simulink model "modele2"  (R2021a)
settings: Solver=VariableStepAuto  StartTime=0.0  StopTime=20  RelTol=10e-8
values from neighbouring files (symbols this model uses):
  A_L = 1    [etablissement_variables.m]
  A_S = 1    [etablissement_variables.m]
  c = 2000.*[1 1 1 1]    [etablissement_variables.m]
  C_x = 1    [etablissement_variables.m]
  Cte_1 = 1    [etablissement_variables.m]
  Cte_2 = 1    [etablissement_variables.m]
  Cte_3 = 1    [etablissement_variables.m]
  Cte_4 = 1    [etablissement_variables.m]
  d_f = 1    [etablissement_variables.m]
  d_r = 1    [etablissement_variables.m]
  g = 9.81    [etablissement_variables.m]
  h = 1    [etablissement_variables.m]
  I = [2 0 0; 0 3 0; 0 0 3]    [etablissement_variables.m]
  J = [1 1 1 1]    [etablissement_variables.m]
  k = 30000.*[1 1 1 1]    [etablissement_variables.m]
  L = l_r+l_f    (= 2)    [etablissement_variables.m]
  l_f = L-l_r    [calcul_N.m]    (also in etablissement_variables.m = 1)
  l_r = 1    [etablissement_variables.m]
  M = 400    [etablissement_variables.m]
  m = M/4.*[l_f/L l_f/L l_r/L l_r/L]    [etablissement_variables.m]
  R = [1 1 1 1]    [etablissement_variables.m]
  rho = 1    [etablissement_variables.m]
undefined symbols (not defined in the file or in its folder): calcul_adherence, calcul_delta, calcul_Fcz, calcul_forceaero, calcul_forces, calcul_forcesprojetees, calcul_lambda, calcul_matriceforces, calcul_matricemoments, calcul_N, calcul_omega, calcul_retourvitesse, calcul_rotaroute, calcul_rotation, calcul_secondterme, calcul_slipangle, calcul_vitessesroues, projection
libraries: dsparch4 x3, slpidlib x2
settings Model: PauseTimes=0.1  Creator=TP-EEA  LastModifiedBy=TP-EEA
settings DebuggingCC: SignalInfNanChecking=error
settings ModelReferenceCC: ModelReferenceMinAlgLoopOccurrences=on

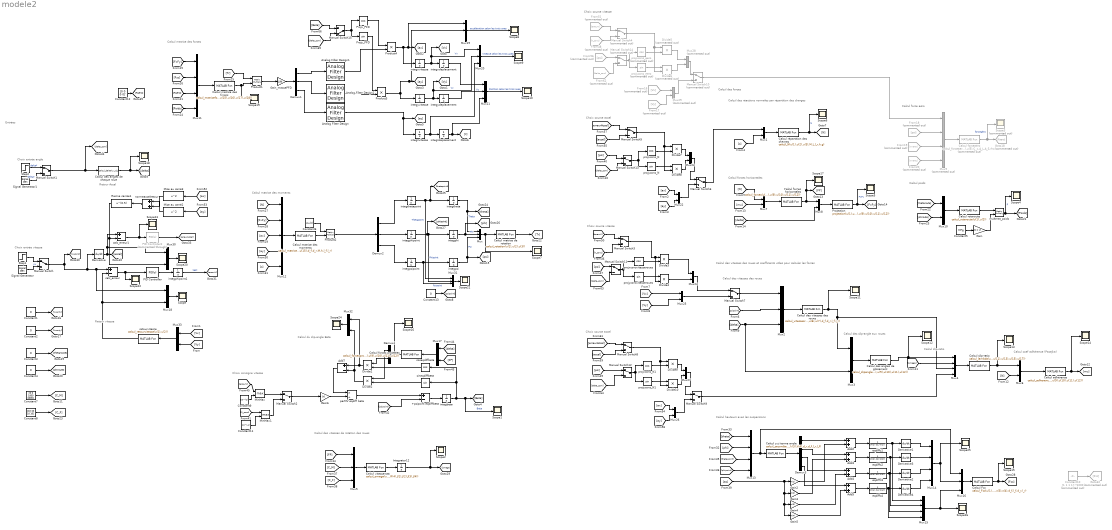
== system modele2 ==
  note: Choix consigne vitesse
  note: Choix entrée vitesse
  note: Choix entrée angle
  note: Choix source accel
  note: Calcul du slip-angle Beta
  note: Calcul des vitesses de rotation des roues
  note: Calcul matrice des forces
  note: Calcul poids
  note: Calcul force aéro
  note: Calcul des forces
  note: Calcul forces horizontales
  note: Calcul des vitesses des roues et coefficients utiles pour calculer les forces
  note: Calcul coef adhérence (Pacejka)
  note: Calcul slip-ratio
  note: Calcul des slip-angle aux roues
  note: Calcul des vitesses des roues
  note: Calcul des réactions normales par répartition des charges
  note: Retour vitesse
  note: Entrées
  note: Calcul matrice des moments
  note: Calcul hauteurs avec les suspensions
  note: Retour Accel
  note: Choix source vitesse
  note: Choix source accel
  note: Choix source vitesse
  +psipoint eqdiffbeta : Sum  Inputs=+-
  Add{2..5} (4 alike) : Sum
  Add7 : Sum  Inputs=+-
  Analog Filter Design : dsparch4/Analog Filter Design  method=Butterworth  filttype=Lowpass  N=4  Wlo=20  Whi=80  Rp=2  Rs=40
  Analog Filter Design1 : dsparch4/Analog Filter Design  method=Butterworth  filttype=Lowpass  N=4  Wlo=20  Whi=80  Rp=2  Rs=40
  Analog Filter Design2 : dsparch4/Analog Filter Design  method=Butterworth  filttype=Lowpass  N=4  Wlo=20  Whi=80  Rp=2  Rs=40
  Calcul Fzc : MATLABFcn  MATLABFcn=calcul_Fcz(u(1),u(2),u(3),u(4),u(5),u(6),u(7),u(8),u(9),u(10),u(11),u(12),k(1),k(2),k(3),k(4),c(1),c(2),c(3),c(4),d_f,l_f,d_r,l_r)  OutputDimensions=4
  Calcul adhérence : MATLABFcn  MATLABFcn=calcul_adherence(u(1),u(2),u(3),u(4),u(5),u(6),u(7),u(8),Cte_1,Cte_2,Cte_3,Cte_4,u(9),u(10),u(11),u(12))  OutputDimensions=4*2
  Calcul des angles de chaque roue : MATLABFcn  MATLABFcn=calcul_delta(u,L,d_f)  OutputDimensions=4
  Calcul des angles de glissement : MATLABFcn  MATLABFcn=calcul_slipangle(u(1),u(2),u(3),u(4),u(5),u(6),u(7),u(8),u(9),u(10),u(11),u(12))  OutputDimensions=4
  Calcul des vitesses des roues : MATLABFcn  MATLABFcn=calcul_vitessesroues(u(1),u(2),u(3),u(4),u(5),u(6),u(7),d_f,d_r,l_f,l_r)  OutputDimensions=4*2
  Calcul forceaéro : MATLABFcn  Commented=on  MATLABFcn=calcul_forceaero(u(1),u(2),u(3),u(4),u(5),C_x,A_L,A_S,rho)  OutputDimensions=3
  Calcul forces horizontales : MATLABFcn  MATLABFcn=calcul_forces(u(1),u(2),u(3),u(4),u(5),u(6),u(7),u(8),u(9),u(10),u(11),u(12))  OutputDimensions=4*2
  Calcul forces projetées : MATLABFcn  MATLABFcn=calcul_forcesprojetees(u(1),u(2),u(3),u(4),u(5),u(6),u(7),u(8),u(9),u(10),u(11),u(12))  OutputDimensions=2  Output1D=off
  Calcul matrice de rotation : MATLABFcn  MATLABFcn=calcul_rotation(u(1),u(2),u(3))  OutputDimensions=[3 3]  Output1D=off
  Calcul matrice des forces : MATLABFcn  MATLABFcn=calcul_matriceforces(u(1),u(2),u(3),u(4),u(5),u(6),u(7),u(8),u(9),u(10),u(11),u(12),u(13),u(14),u(15),u(16),u(17),u(18))  OutputDimensions=[3 1]  Output1D=off
  Calcul matrice des moments : MATLABFcn  MATLABFcn=calcul_matricemoments(u(1),u(2),u(3),u(4),u(5),u(6),u(7),u(8),u(9),u(10),u(11),u(12),u(13),u(14),u(15),d_f,d_r,M,h,l_f,l_r)  OutputDimensions=[3 1]  Output1D=off
  Calcul rotaroute : MATLABFcn  MATLABFcn=calcul_rotaroute(u(1),u(2))  OutputDimensions=[3 3]  Output1D=off
  Calcul répartition des charges : MATLABFcn  MATLABFcn=calcul_N(u(1),u(2),u(3),M,L,l_r,h,g)  OutputDimensions=4
  Calcul slip-ratio : MATLABFcn  MATLABFcn=calcul_lambda(u(1),u(2),u(3),u(4),R(1),R(2),R(3),R(4),u(5),u(6),u(7),u(8),u(9),u(11),u(13),u(15),u(17))  OutputDimensions=4*2
  Calcul vitesserota : MATLABFcn  MATLABFcn=calcul_omega(u(1),u(2),u(3),u(4),u(5),u(6),u(7),u(8),u(9),u(10),u(11),u(12),u(13),u(14),u(15),u(16),R(1),R(2),R(3),R(4),J(1),J(2),J(3),J(4))  OutputDimensions=4
  Calcul z-zi terme angle : MATLABFcn  MATLABFcn=calcul_secondterme(u(1),u(2),u(3),u(4),c(1),c(2),c(3),c(4),k(1),k(2),k(3),k(4),d_r,d_f,l_r,l_f)  OutputDimensions=4
  Constant{1..4,13} (5 alike) : Constant  Value=0
  Constant10 : Constant  Commented=on  Value=[1 1 1 1]'.*1000  VectorParams1D=off
  Constant11 : Constant  Value=10^(-1)
  Constant12 : Constant  Value=[0 0 0 0]'
  Constant5 : Constant  Value=M*g  VectorParams1D=off
  Constant6 : Constant  Value=inv(I)
  Constant7 : Constant  Value=[0 0 1000 1000]
  Constant8 : Constant  Value=[10 10 10 10]
  Constant9 : Constant  Value=10^(-1)
  Demux1 : Demux  Outputs=3
  Demux2 : Demux  Outputs=3
  Demux3 : Demux
  Demux4 : Demux  Outputs=2
  Derivative{,1..4} (5 alike) : Derivative
  Divide{1..4,7..10} (8 alike) : Product  Inputs=**
  Divide5 : Product  Commented=on  Inputs=**
  Divide6 : Product  Commented=on  Inputs=**
  From16 : From  Commented=on  GotoTag=Vx
  From17 : From  Commented=on  GotoTag=Vy
  From18 : From  Commented=on  GotoTag=psi
  From19 : From  Commented=on  GotoTag=Vventx
  From20 : From  Commented=on  GotoTag=Vventy
  From48 : From  Commented=on  GotoTag=V_cons
  From51 : From  Commented=on  GotoTag=erreurV
  From56 : From  Commented=on  GotoTag=psi
  From62 : From  Commented=on  GotoTag=delta_com
  Gain : Gain  Gain=[0 0 1]'
  Gain2 : Gain  Gain=m(1)
  Gain3 : Gain  Gain=m(2)
  Gain4 : Gain  Gain=m(3)
  Gain5 : Gain  Gain=m(4)
  Gain6 : Gain  Gain=M
  Gain_massePFD : Gain  Gain=1/M
  Goto18 : Goto  Commented=on  GotoTag=Faero
  Goto32 : Goto  Commented=on  GotoTag=Fzc
  Integrator12 : Integrator
  Manual Switch{,1..3,5..9,11..13} (12 alike) : ManualSwitch
  Manual Switch10 : ManualSwitch  Commented=on
  Manual Switch14 : ManualSwitch  Commented=on
  Manual Switch15 : ManualSwitch  CurrentSetting=0
  Manual Switch4 : ManualSwitch  Commented=on
  MinMax : MinMax  Function=max  Inputs=2
  MinMax1 : MinMax  Function=max  Inputs=2
  Mise au carré2 : MATLABFcn  MATLABFcn=u^2
  Mise au carré3 : MATLABFcn  MATLABFcn=u^2
  Mux{,2,5,16,19..21,31} (8 alike) : Mux  Inputs=3
  Mux{1,3,6..8,10,17..18,22..27,30,32..33} (17 alike) : Mux  Inputs=2
  Mux{4,11,13..15} (5 alike) : Mux
  Mux12 : Mux  Inputs=5
  Mux28 : Mux  Commented=on  Inputs=2
  Mux29 : Mux  Commented=on  Inputs=2
  Mux9 : Mux  Commented=on
  PID Controller : slpidlib/PID Controller  Controller=PID  Form=Parallel  TimeDomain=Continuous-time  UseExternalTs=off  SampleTime=-1  IntegratorMethod=Forward Euler  FilterMethod=Forward Euler  ControllerParametersSource=internal  P=1  I=1000  D=0  UseFilter=on  N=100  TunerSelectOption=Transfer Function Based (PID Tuner App)  InitialConditionSource=internal  InitialConditionForIntegrator=0  InitialConditionForFilter=0  DifferentiatorICPrevScaledInput=0  ExternalReset=none  TrackingMode=off  Kt=1  LimitOutput=off  SatLimitsSource=internal  UpperSaturationLimit=inf  LowerSaturationLimit=-inf  LinearizeAsGain=on  AntiWindupMode=none  Kb=1  POutMin=[]  POutMax=[]  IOutMin=[]  IOutMax=[]  DOutMin=[]  DOutMax=[]  NOutMin=[]  NOutMax=[]  SumOutMin=[]  SumOutMax=[]  SaturationOutMin=[]  SaturationOutMax=[]  PParamMin=[]  PParamMax=[]  IParamMin=[]  IParamMax=[]  DParamMin=[]  DParamMax=[]  NParamMin=[]  NParamMax=[]  KbParamMin=[]  KbParamMax=[]  KtParamMin=[]  KtParamMax=[]  KbOutMin=[]  KbOutMax=[]  KtOutMin=[]  KtOutMax=[]  IntegratorOutMin=[]  IntegratorOutMax=[]  FilterOutMin=[]  FilterOutMax=[]  SumI1OutMin=[]  SumI1OutMax=[]  SumI2OutMin=[]  SumI2OutMax=[]  SumI3OutMin=[]  SumI3OutMax=[]  SumI4OutMin=[]  SumI4OutMax=[]  SumDOutMin=[]  SumDOutMax=[]  DifferentiatorOutMin=[]  DifferentiatorOutMax=[]  FilterDiffOutCoefMin=[]  FilterDiffOutCoefMax=[]  ReciprocalOutMin=[]  ReciprocalOutMax=[]  SumDenOutMin=[]  SumDenOutMax=[]  SumNumOutMin=[]  SumNumOutMax=[]  DivideOutMin=[]  DivideOutMax=[]  UdiffTsProdOutMin=[]  UdiffTsProdOutMax=[]  NTsProdOutMin=[]  NTsProdOutMax=[]  UintegralTsProdOutMin=[]  UintegralTsProdOutMax=[]  UngainTsProdOutMin=[]  UngainTsProdOutMax=[]  IntegratorContinuousStateAttributes=''  IntegratorStateMustResolveToSignalObject=off  IntegratorRTWStateStorageClass=Auto  FilterContinuousStateAttributes=''  FilterStateMustResolveToSignalObject=off  FilterRTWStateStorageClass=Auto  ParallelPVariant=InternalParameters  IdealPVariant=Disabled  IVariant=InternalParameters  DVariant=InternalParameters  IntegratorVariant=Continuous  SatVariant=Disabled  AWVariant=Passthrough  PCopyVariant=Disabled  TRVariant=Disabled  FdbkBlocksVariant=Forward  IdealPFdbkVariant=Disabled  SatFdbkVariant=Disabled  DerivativeFilterVariant=ContFilter  NVariant=InternalParameters  NCopyVariant=Disabled  FilterICVariant=InternalICsFilter  IntegratorICVariant=InternalICs  ExternalResetVariant=Disabled  TRSumVariant=Passthrough  SumFdbkVariant=Disabled  SumVariant=Sum_PID  TsampFilterVariant=InternalTs  TsampNgainVariant=Passthrough  TsampIntegralVariant=Passthrough  ExternalSaturationOutDataTypeStr=Inherit: Same as second input
  PID Controller2 : slpidlib/PID Controller  Commented=through  Controller=PID  Form=Parallel  TimeDomain=Continuous-time  UseExternalTs=off  SampleTime=-1  IntegratorMethod=Forward Euler  FilterMethod=Forward Euler  ControllerParametersSource=internal  P=1  I=1  D=0  UseFilter=on  N=100  TunerSelectOption=Transfer Function Based (PID Tuner App)  InitialConditionSource=internal  InitialConditionForIntegrator=0  InitialConditionForFilter=0  DifferentiatorICPrevScaledInput=0  ExternalReset=none  TrackingMode=off  Kt=1  LimitOutput=off  SatLimitsSource=internal  UpperSaturationLimit=inf  LowerSaturationLimit=-inf  LinearizeAsGain=on  AntiWindupMode=none  Kb=1  POutMin=[]  POutMax=[]  IOutMin=[]  IOutMax=[]  DOutMin=[]  DOutMax=[]  NOutMin=[]  NOutMax=[]  SumOutMin=[]  SumOutMax=[]  SaturationOutMin=[]  SaturationOutMax=[]  PParamMin=[]  PParamMax=[]  IParamMin=[]  IParamMax=[]  DParamMin=[]  DParamMax=[]  NParamMin=[]  NParamMax=[]  KbParamMin=[]  KbParamMax=[]  KtParamMin=[]  KtParamMax=[]  KbOutMin=[]  KbOutMax=[]  KtOutMin=[]  KtOutMax=[]  IntegratorOutMin=[]  IntegratorOutMax=[]  FilterOutMin=[]  FilterOutMax=[]  SumI1OutMin=[]  SumI1OutMax=[]  SumI2OutMin=[]  SumI2OutMax=[]  SumI3OutMin=[]  SumI3OutMax=[]  SumI4OutMin=[]  SumI4OutMax=[]  SumDOutMin=[]  SumDOutMax=[]  DifferentiatorOutMin=[]  DifferentiatorOutMax=[]  FilterDiffOutCoefMin=[]  FilterDiffOutCoefMax=[]  ReciprocalOutMin=[]  ReciprocalOutMax=[]  SumDenOutMin=[]  SumDenOutMax=[]  SumNumOutMin=[]  SumNumOutMax=[]  DivideOutMin=[]  DivideOutMax=[]  UdiffTsProdOutMin=[]  UdiffTsProdOutMax=[]  NTsProdOutMin=[]  NTsProdOutMax=[]  UintegralTsProdOutMin=[]  UintegralTsProdOutMax=[]  UngainTsProdOutMin=[]  UngainTsProdOutMax=[]  IntegratorContinuousStateAttributes=''  IntegratorStateMustResolveToSignalObject=off  IntegratorRTWStateStorageClass=Auto  FilterContinuousStateAttributes=''  FilterStateMustResolveToSignalObject=off  FilterRTWStateStorageClass=Auto  ParallelPVariant=InternalParameters  IdealPVariant=Disabled  IVariant=InternalParameters  DVariant=InternalParameters  IntegratorVariant=Continuous  SatVariant=Disabled  AWVariant=Passthrough  PCopyVariant=Disabled  TRVariant=Disabled  FdbkBlocksVariant=Forward  IdealPFdbkVariant=Disabled  SatFdbkVariant=Disabled  DerivativeFilterVariant=ContFilter  NVariant=InternalParameters  NCopyVariant=Disabled  FilterICVariant=InternalICsFilter  IntegratorICVariant=InternalICs  ExternalResetVariant=Disabled  TRSumVariant=Passthrough  SumFdbkVariant=Disabled  SumVariant=Sum_PID  TsampFilterVariant=InternalTs  TsampNgainVariant=Passthrough  TsampIntegralVariant=Passthrough  ExternalSaturationOutDataTypeStr=Inherit: Same as second input
  Product1 : Product  Multiplication=Matrix(*)
  Product2 : Product  Multiplication=Matrix(*)
  Product3 : Product
  Product4 : Product
  Projection : MATLABFcn  MATLABFcn=projection(u(1),u(2),u(3),u(4),u(5),u(6),u(7),u(8),u(9),u(10),u(11),u(12))  OutputDimensions=8
  Projx_PFD : Trigonometry  Operator=cos
  Projy_PFD : Trigonometry
  Racine carrée1 : MATLABFcn  MATLABFcn=u^(0.5)
  Scope{,1..2,4..26} (26 alike) : Scope
  Scope3 : Scope  Commented=on
  Signal Generator : SignalGenerator  Frequency=0.1  Units=rad/sec
  Signal Generator1 : SignalGenerator  Frequency=0.01  Units=rad/sec
  Step1 : Step  Time=0  After=10/3.6  SampleTime=0
  Step2 : Step  Time=0  After=0  SampleTime=0
  calc_erreur : Sum  Inputs=+-
  calc_erreur1 : Sum  Inputs=+-
  coseqdiffbeta : Trigonometry  Operator=cos
  eqdiffz1 : TransferFcn  Denominator=[m(1) c(1) k(1)]
  eqdiffz2 : TransferFcn  Denominator=[m(2) c(2) k(2)]
  eqdiffz3 : TransferFcn  Denominator=[m(3) c(3) k(3)]
  eqdiffz4 : TransferFcn  Denominator=[m(4) c(4) k(4)]
  integbeta : Integrator
  integphi : Integrator
  integphipoint : Integrator
  integphipoint1 : Integrator
  integpsi : Integrator
  integpsipoint : Integrator
  integtheta : Integrator
  integthetapoint : Integrator  InitialCondition=0.01
  integxdeplacement : Integrator
  integxvitesse : Integrator
  integydeplacement : Integrator
  integyvitesse : Integrator
  integzdeplacement : Integrator
  integzvitesse : Integrator
  multmat_poids : Product  Multiplication=Matrix(*)
  normeaccelretour : Sum
  parMV eqdiff beta : Product  Inputs=*/
  projxcons_N : Trigonometry  Operator=cos
  projxcons_N1 : Trigonometry  Operator=cos
  projxcons_aero : Trigonometry  Commented=on  Operator=cos
  projxconsvitesseroues : Trigonometry  Operator=cos
  projycons_N : Trigonometry
  projycons_N1 : Trigonometry
  projycons_aero : Trigonometry  Commented=on
  projyconsvitesseroues : Trigonometry
  retourvitesse : MATLABFcn  MATLABFcn=calcul_retourvitesse(u(1),u(2))  OutputDimensions=1
  sineqdiffbeta : Trigonometry
  wires:
  integxvitesse/1 -> Mux20/1, [Vx], integxdeplacement/1  "Vx"
  integyvitesse/1 -> Mux20/2, [Vy], integydeplacement/1  "Vy"
  integthetapoint/1 -> Mux31/1, [thetapoint], integtheta/1  "Thetapoint"
  integzvitesse/1 -> Mux20/3, integzdeplacement/1  "Vz"
  integpsipoint/1 -> Mux31/3, integpsi/1  "Psipoint"
  integphipoint/1 -> Mux31/2, integphi/1, [phipoint]  "Phipoint"
  integtheta/1 -> [theta], Mux/1  "Theta"
  integphi/1 -> [phi], Mux/2  "Phi"
  integpsi/1 -> Mux/3, [psi]  "Psi"
  [Vx] -> Mux33/1
  [Vy] -> Mux33/2
  retourvitesse/1 -> calc_erreur/2, Mux18/2
  integzdeplacement/1 -> Mux21/3, [z]
  Mux1/1 -> Calcul répartition des charges/1
  Calcul répartition des charges/1 -> Scope6/1, [N]  "N"
  Mux2/1 -> Calcul des vitesses des roues/1
  [delta] -> Mux3/2, Mux2/3
  Calcul des vitesses des roues/1 -> Scope11/1, Mux4/3, Mux3/1
  Mux3/1 -> Calcul des angles de glissement/1
  Manual Switch9/1 -> Mux4/4
  [omega] -> Mux4/2
  Mux4/1 -> Calcul slip-ratio/1
  Mux6/1 -> Calcul adhérence/1
  Calcul slip-ratio/1 -> Scope13/1, Mux6/1
  [N] -> Mux6/2
  Calcul adhérence/1 -> Scope14/1, [mu]
  [N] -> Mux7/1
  [mu] -> Mux7/2
  Mux7/1 -> Calcul forces horizontales/1
  Mux8/1 -> Projection/1
  [delta] -> Mux8/2
  Calcul forces horizontales/1 -> Scope17/1, [FP], Mux8/1
  Projection/1 -> Scope5/1, [FxFy]  "FxFy"
  Constant1/1 -> [Vventx]
  Constant2/1 -> [Vventy]
  From20/1 -> Mux9/4
  Mux9/1 -> Calcul forceaéro/1
  Calcul forceaéro/1 -> Scope3/1, Goto18/1  "forceaéro"
  Constant3/1 -> [thetaroute]
  Constant4/1 -> [phiroute]
  [thetaroute] -> Mux10/1
  [phiroute] -> Mux10/2
  Mux10/1 -> Calcul rotaroute/1
  Calcul rotaroute/1 -> multmat_poids/1
  Constant5/1 -> Gain/1
  Gain/1 -> multmat_poids/2
  multmat_poids/1 -> Scope4/1, [Poids]  "P"
  Calcul matrice de rotation/1 -> [Tr]
  Mux11/1 -> Calcul matrice des forces/1
  [FxFy] -> Mux11/1
  [Fzc] -> Mux11/2
  [Faero] -> Mux11/3
  [Poids] -> Mux11/4
  [Tr] -> Product1/1
  Calcul matrice des forces/1 -> Scope19/1, Product1/2
  Product1/1 -> Gain_massePFD/1
  [N] -> Mux12/1
  [FxFy] -> Mux12/2
  [ax] -> Mux12/3
  [ay] -> Mux12/4
  [z] -> Mux12/5
  Mux12/1 -> Calcul matrice des moments/1
  Calcul matrice des moments/1 -> Product2/2
  Constant6/1 -> Product2/1
  Product2/1 -> Demux2/1
  Demux2/1 -> integthetapoint/1
  Demux2/2 -> integphipoint/1
  Demux2/3 -> integpsipoint/1
  Mux13/1 -> Mux16/1, Calcul z-zi terme angle/1
  [theta] -> Mux13/1
  [phi] -> Mux13/2
  [thetapoint] -> Mux13/3
  [phipoint] -> Mux13/4
  [az] -> Gain5/1, Gain4/1, Gain3/1, Gain2/1
  Calcul z-zi terme angle/1 -> Demux3/1
  Demux3/1 -> Add2/1
  Gain2/1 -> Add2/2
  Demux3/2 -> Add3/1
  Gain3/1 -> Add3/2
  Demux3/3 -> Add4/1
  Gain4/1 -> Add4/2
  Demux3/4 -> Add5/1
  Gain5/1 -> Add5/2
  Add2/1 -> eqdiffz1/1
  Add3/1 -> eqdiffz2/1
  Add4/1 -> eqdiffz3/1
  Add5/1 -> eqdiffz4/1
  eqdiffz1/1 -> Mux15/1, Derivative1/1
  eqdiffz2/1 -> Mux15/2, Derivative3/1
  eqdiffz3/1 -> Mux15/3, Derivative2/1
  eqdiffz4/1 -> Mux15/4, Derivative4/1
  Derivative1/1 -> Mux14/1
  Derivative3/1 -> Mux14/2
  Derivative2/1 -> Mux14/3
  Derivative4/1 -> Mux14/4
  Mux14/1 -> Scope25/1, Mux16/2
  Mux15/1 -> Scope26/1, Mux16/3
  Mux16/1 -> Calcul Fzc/1
  Constant7/1 -> [C_M]
  Constant8/1 -> [C_F]
  [FP] -> Mux5/1
  [C_M] -> Mux5/2
  [C_F] -> Mux5/3
  Mux5/1 -> Calcul vitesserota/1
  Calcul vitesserota/1 -> Integrator12/1
  Product4/1 -> integxvitesse/1, Mux19/1, [ax]
  Product3/1 -> Mux19/2, [ay], integyvitesse/1
  integbeta/1 -> coseqdiffbeta/1, sineqdiffbeta/1, Scope1/1, [Beta]  "Beta"
  +psipoint eqdiffbeta/1 -> integbeta/1
  Gain6/1 -> parMV eqdiff beta/2
  parMV eqdiff beta/1 -> +psipoint eqdiffbeta/1
  Mux17/1 -> Calcul forces projetées/1
  [delta] -> Mux17/1
  [FP] -> Mux17/2
  Calcul forces projetées/1 -> Scope16/1, Demux4/1
  Demux4/2 -> Divide1/1
  coseqdiffbeta/1 -> Divide1/2
  Divide1/1 -> Mux32/1, Add7/1
  Demux4/1 -> Divide2/1
  sineqdiffbeta/1 -> Divide2/2
  Divide2/1 -> Mux32/2, Add7/2
  Add7/1 -> parMV eqdiff beta/1
  Constant9/1 -> MinMax/2
  Mux18/1 -> Scope/1
  [erreurV] -> MinMax/1
  projxconsvitesseroues/1 -> Divide3/2
  projyconsvitesseroues/1 -> Divide4/1
  Mux19/1 -> Scope8/1  "accélération selon les trois axes"
  Mux20/1 -> Scope9/1  "Vitesse selon les trois axes"
  Mux21/1 -> Scope10/1  "Position selon les trois axes"
  integxdeplacement/1 -> Mux21/1
  integydeplacement/1 -> Mux21/2
  Calcul des angles de glissement/1 -> Scope12/1, Mux4/1
  Signal Generator/1 -> Manual Switch/2  "V*"
  Manual Switch/1 -> [V_cons], Derivative/1, Mux18/1, calc_erreur/1
  Step1/1 -> Manual Switch/1
  Step2/1 -> Manual Switch1/1  "delta*"
  Signal Generator1/1 -> Manual Switch1/2  "delta*"
  MinMax/1 -> Manual Switch2/1
  Manual Switch2/1 -> Gain6/1
  projycons_aero/1 -> Divide6/1
  projxcons_aero/1 -> Divide5/2
  [V_cons] -> Manual Switch3/2
  Manual Switch3/1 -> Divide4/2, Divide3/1
  From48/1 -> Manual Switch4/2
  Manual Switch4/1 -> Divide6/2, Divide5/1
  Mise au carré2/1 -> normeaccelretour/1
  [ay] -> Mise au carré2/1
  Mise au carré3/1 -> normeaccelretour/2
  [ax] -> Mise au carré3/1
  normeaccelretour/1 -> Racine carrée1/1
  [accel] -> Manual Switch5/2
  Manual Switch5/1 -> Divide8/2, Divide7/1
  projxcons_N/1 -> Divide7/2
  [erreurAccel] -> Manual Switch5/1
  projycons_N/1 -> Divide8/1
  Mux23/1 -> Manual Switch6/1
  Divide7/1 -> Mux23/1
  Divide8/1 -> Mux23/2
  [ax] -> Mux22/1
  [ay] -> Mux22/2
  Mux22/1 -> Manual Switch6/2
  Manual Switch6/1 -> Mux1/1
  Divide4/1 -> Mux24/2
  Mux24/1 -> Manual Switch7/1
  Divide3/1 -> Mux24/1
  Mux25/1 -> Manual Switch7/2
  [psipoint] -> Mux2/2
  Manual Switch7/1 -> Mux2/1
  [Vy] -> Mux25/2
  [Vx] -> Mux25/1
  Divide9/1 -> Mux27/1
  Manual Switch8/1 -> Divide10/2, Divide9/1
  Mux27/1 -> Manual Switch9/1
  [accel] -> Manual Switch8/2
  [ax] -> Mux26/1
  projycons_N1/1 -> Divide10/1
  Divide10/1 -> Mux27/2
  projxcons_N1/1 -> Divide9/2
  [erreurAccel] -> Manual Switch8/1
  Mux26/1 -> Manual Switch9/2
  [ay] -> Mux26/2
  From19/1 -> Mux9/3
  Manual Switch10/1 -> Mux9/1
  Mux29/1 -> Manual Switch10/2
  From16/1 -> Mux29/1
  From17/1 -> Mux29/2
  Divide5/1 -> Mux28/1
  Divide6/1 -> Mux28/2
  Calcul des angles de chaque roue/1 -> Scope18/1, [delta]
  Manual Switch1/1 -> [delta_com], Calcul des angles de chaque roue/1
  Constant11/1 -> MinMax1/2
  [V_cons] -> MinMax1/1
  MinMax1/1 -> Manual Switch2/2
  [z] -> Mux1/2
  From18/1 -> Mux9/2
  Racine carrée1/1 -> Mux30/2, calc_erreur1/2
  Mux30/1 -> Scope20/1
  Derivative/1 -> Mux30/1, calc_erreur1/1, [accel]
  Mux28/1 -> Manual Switch10/1
  Mux/1 -> Scope7/1, Calcul matrice de rotation/1
  [psipoint] -> +psipoint eqdiffbeta/2
  Mux31/1 -> Scope21/1
  Projy_PFD/1 -> Product3/1
  Gain_massePFD/1 -> Demux1/1
  Demux1/3 -> Analog Filter Design/1
  Analog Filter Design/1 -> integzvitesse/1, [az]
  Demux1/2 -> Analog Filter Design2/1
  Analog Filter Design2/1 -> Product3/2
  Analog Filter Design1/1 -> Product4/2
  Demux1/1 -> Analog Filter Design1/1
  calc_erreur/1 -> PID Controller/1, Scope22/1
  PID Controller/1 -> integphipoint1/1
  calc_erreur1/1 -> Scope23/1, PID Controller2/1
  PID Controller2/1 -> [erreurAccel]
  Constant10/1 -> Goto32/1
  [erreurV] -> Manual Switch3/1
  From51/1 -> Manual Switch4/1
  Mux32/1 -> Scope24/1
  [psi] -> Manual Switch11/1
  [delta_com] -> Manual Switch11/2
  Manual Switch11/1 -> projyconsvitesseroues/1, projxconsvitesseroues/1
  [psi] -> Manual Switch12/1
  [delta_com] -> Manual Switch12/2
  Manual Switch12/1 -> projycons_N1/1, projxcons_N1/1
  Manual Switch13/1 -> projycons_N/1, projxcons_N/1
  [psi] -> Manual Switch13/1
  [delta_com] -> Manual Switch13/2
  Manual Switch14/1 -> projycons_aero/1, projxcons_aero/1
  From56/1 -> Manual Switch14/1
  From62/1 -> Manual Switch14/2
  Manual Switch15/1 -> Projy_PFD/1, Projx_PFD/1
  [Beta] -> Manual Switch15/1
  [delta_com] -> Manual Switch15/2
  Projx_PFD/1 -> Product4/1
  Integrator12/1 -> Scope2/1, [omega]
  Constant12/1 -> [Faero]
  Mux33/1 -> retourvitesse/1
  Calcul Fzc/1 -> [Fzc], Scope15/1
  Constant13/1 -> [psipoint]
  integphipoint1/1 -> [erreurV]  "test"
